simulink model "lagrange_model"  (R2022a)
settings: Solver=ode4  StartTime=0.0  StopTime=10.0  FixedStep=0.01  RelTol=1e-3
undefined symbols (not defined in the file or in its folder): DiscIntNeverNeededParam
(part 1 of 5)
settings Model: Creator=legacy  LastModifiedBy=legacy

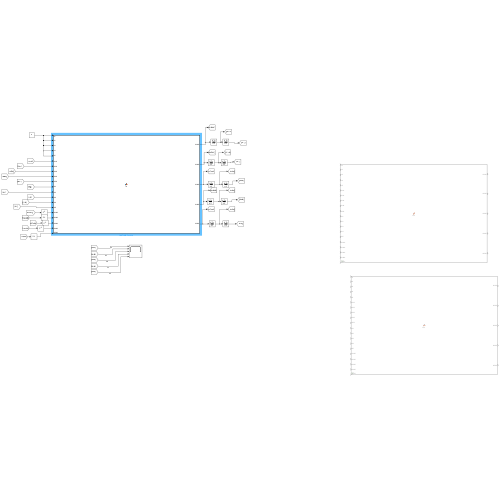
[thumbnail: Simulink's stored preview of the top-level diagram]
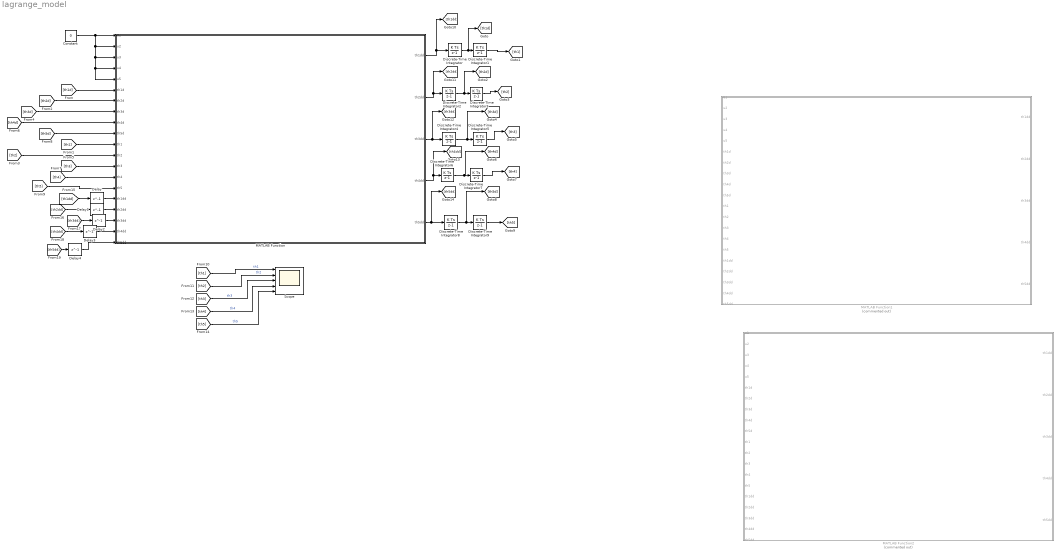
== system lagrange_model ==
  Constant : Constant  Value=0
  Delay{,1..4} (5 alike) : Delay  DelayLength=1  SampleTime=0.01
  Discrete-Time Integrator{,1..9} (10 alike) : DiscreteIntegrator  SampleTime=0.01  ICPrevOutput=DiscIntNeverNeededParam  ICPrevScaledInput=DiscIntNeverNeededParam
  MATLAB Function : MATLAB Function  TreatAsAtomicUnit=on
  MATLAB Function1 : MATLAB Function  Commented=on  TreatAsAtomicUnit=on
  MATLAB Function2 : MATLAB Function  Commented=on  TreatAsAtomicUnit=on
  Scope : Scope  NumInputPorts=5
  wires:
  MATLAB Function/1(th1dd) -> Discrete-Time Integrator/1, [th1dd]
  MATLAB Function/3(th3dd) -> Discrete-Time Integrator4/1, [th3dd]
  MATLAB Function/5(th5dd) -> Discrete-Time Integrator8/1, [th5dd]
  Discrete-Time Integrator3/1 -> [th2]
  Discrete-Time Integrator5/1 -> [th3]
  Discrete-Time Integrator7/1 -> [th4]
  [th1d] -> MATLAB Function/6(th1d)
  [th2d] -> MATLAB Function/7(th2d)
  [th3d] -> MATLAB Function/8(th3d)
  [th4d] -> MATLAB Function/9(th4d)
  [th5d] -> MATLAB Function/10(th5d)
  [th1] -> MATLAB Function/11(th1)
  [th2] -> MATLAB Function/12(th2)
  [th3] -> MATLAB Function/13(th3)
  [th4] -> MATLAB Function/14(th4)
  [th5] -> MATLAB Function/15(th5)
  [th1] -> Scope/1  "th1"
  [th2] -> Scope/2  "th2"
  [th3] -> Scope/3  "th3"
  [th4] -> Scope/4  "th4"
  [th5] -> Scope/5  "th5"
  Constant/1 -> MATLAB Function/5(u5), MATLAB Function/4(u4), MATLAB Function/3(u3), MATLAB Function/2(u2), MATLAB Function/1(u1)
  Discrete-Time Integrator/1 -> [th1d], Discrete-Time Integrator1/1
  Discrete-Time Integrator1/1 -> [th1]
  Discrete-Time Integrator2/1 -> [th2d], Discrete-Time Integrator3/1
  MATLAB Function/2(th2dd) -> [th2dd], Discrete-Time Integrator2/1
  Discrete-Time Integrator4/1 -> [th3d], Discrete-Time Integrator5/1
  Discrete-Time Integrator6/1 -> [th4d], Discrete-Time Integrator7/1
  MATLAB Function/4(th4dd) -> [th4dd], Discrete-Time Integrator6/1
  Discrete-Time Integrator8/1 -> [th5d], Discrete-Time Integrator9/1
  Discrete-Time Integrator9/1 -> [th5]
  [th1dd] -> Delay/1
  [th2dd] -> Delay1/1
  [th3dd] -> Delay2/1
  [th4dd] -> Delay3/1
  [th5dd] -> Delay4/1
  Delay/1 -> MATLAB Function/16("th1dd ")
  Delay1/1 -> MATLAB Function/17("th2dd ")
  Delay2/1 -> MATLAB Function/18("th3dd ")
  Delay3/1 -> MATLAB Function/19("th4dd ")
  Delay4/1 -> MATLAB Function/20("th5dd ")
